simulink model "assignment_project_onclass_observerp"  (R2022a)
settings: Solver=VariableStepAuto  StartTime=0.0  StopTime=100  FixedStep=0.001  RelTol=1e-3
values from neighbouring files (symbols this model uses):
  A_LD = [  -skew(Oc),    eye(3),          -skew(Vc),      zeros(3),      zeros(3,4) ... (first row only)    [project_disturbance_observer.m]
  B_LD = [    [0;0;0],     zeros(3) ... (first row only)    [project_disturbance_observer.m]
  C_LD = [eye(3),zeros(3),zeros(3),zeros(3),zeros(3,4) ... (first row only)    [project_disturbance_observer.m]
  K = lqr(A, B, Q, R)    [Linear_model.m]    (also in project_disturbance_observer.m = lqr(A_LD,B_LD,Q,R))
undefined symbols (not defined in the file or in its folder): L
libraries: robotcorelib x1, uavutilslib x1
settings Model: PacingRate=5  Creator=yulinchen  LastModifiedBy=FLKU
settings SolverCC: AlgebraicLoopSolver=TrustRegion
settings DebuggingCC: SFMachineParentedDataDiag=warning
settings ModelReferenceCC: EnableRefExpFcnMdlSchedulingChecks=off
settings RTWCC: Description=Generic Real-Time Target

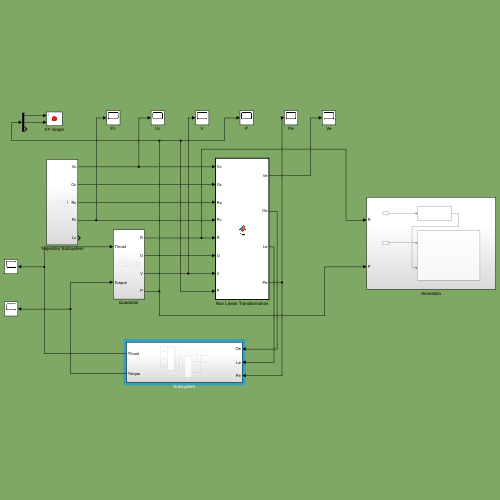
[thumbnail: Simulink's stored preview of the top-level diagram]
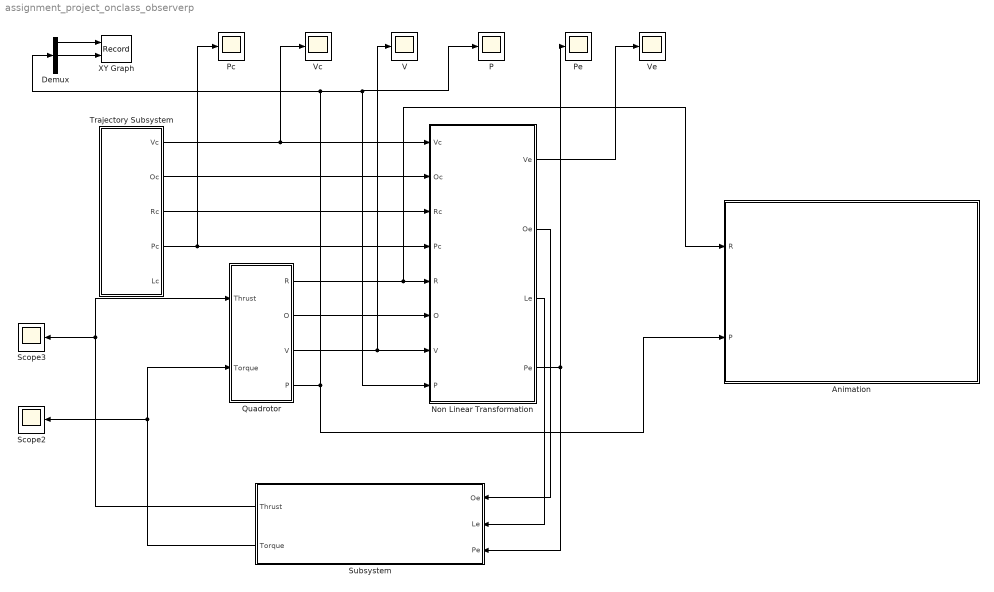
== system assignment_project_onclass_observerp ==
  Animation : Subsystem
  Demux : Demux  Outputs=3
  Non Linear Transformation : MATLAB Function  TreatAsAtomicUnit=on
  P : Scope
  Pc : Scope
  Pe : Scope
  Quadrotor : Subsystem
  Scope2 : Scope
  Scope3 : Scope
  Subsystem : Subsystem
  Trajectory Subsystem : Subsystem
  V : Scope
  Vc : Scope
  Ve : Scope
  XY Graph : Record  FileSettingsInternal="{\"entries\":[{\"content\":{\"excelSettings\":{\"content\":{},\"type\":\"Streamout.ExcelSettings\"}},\"type\":\"Streamout.FileSettingStorage\",\"uuid\":\"d99a883c-f2c1-4db8-87d8-b50552af1765\"}],\"packageUris\":[\"http://schema.mathworks.com/mf0/streamout_blocks/R2020a\"],\"version\":\"1.0\"}"  Layout=[1 1]  SignalsInternal="{\"entries\":[{\"content\":{\"signals\":[{\"content\":{\"blockPath\":[\"assignment_project_onclass_observerp/XY Graph\"],\"channel\":[],\"dimensions\":[1],\"domain\":\"assignment_project_onclass_observerp/XY Graph\",\"lineColor\":\"#a2142f\",\"plots\":[1],\"port\":1,\"sid\":[\"\"],\"signalID\":262,\"signalName\":\"Demux:1\"},\"type\":\"RecordBlkView.Signal\",\"uuid\":\"ec450a59-525e-442a-974f-52693ac6a144\"},{\"content\":{\"blockPath\":[\"assignment_project_onclass_observerp/XY Graph\"],\"channel\":[],\"dimensions\":[1],\"domain\":\"assignment_project_onclass_observerp/XY Graph\",\"lineColor\":\"#139fff\",\"plots\":[1],\"port\":2,\"sid\":[\"\"],\"signalID\":266,\"signalName\":\"Demux:2\"},\"type\":\"RecordBlkView.Signal\",\"uuid\":\"cccf172e-75eb-4d21-8fee-72d7a7188919\"}]},\"type\":\"RecordBlkView.InputSignals\",\"uuid\":\"7c770795-19c4-4b78-8178-cc713b2e03cc\"}],\"packageUris\":[\"http://schema.mathworks.com/mf0/streamout_blocks/R2020a\"],\"version\":\"1.0\"}"  VisualizationBindings="{\"xyplotplugin\":{\"info\":[{\"series\":[{\"bindingParametersList\":[{\"parameter\":\"X-Axis\",\"signalID\":262,\"signalName\":\"Demux:1\"},{\"parameter\":\"Y-Axis\",\"signalID\":266,\"signalName\":\"Demux:2\"}],\"seriesID\":13484}],\"subplotID\":1}]}}"  CompatibilityTag=XY  st=-1
  wires:
  Trajectory Subsystem/1(Vc) -> Vc/1, Non Linear Transformation/1(Vc)
  Trajectory Subsystem/2(Oc) -> Non Linear Transformation/2(Oc)
  Trajectory Subsystem/3(Rc) -> Non Linear Transformation/3(Rc)
  Trajectory Subsystem/4(Pc) -> Pc/1, Non Linear Transformation/4(Pc)
  Quadrotor/1(R) -> Animation/1(R), Non Linear Transformation/5(R)
  Quadrotor/2(O) -> Non Linear Transformation/6(O)
  Quadrotor/3(V) -> V/1, Non Linear Transformation/7(V)
  Quadrotor/4(P) -> Animation/2(P), Demux/1, Non Linear Transformation/8(P), P/1
  Non Linear Transformation/1(Ve) -> Ve/1
  Demux/1 -> XY Graph/1
  Non Linear Transformation/4(Pe) -> Pe/1, Subsystem/3(Pe)
  Subsystem/1(Thrust) -> Quadrotor/1(Thrust), Scope3/1
  Subsystem/2(Torque) -> Quadrotor/2(Torque), Scope2/1
  Non Linear Transformation/2(Oe) -> Subsystem/1(Oe)
  Non Linear Transformation/3(Le) -> Subsystem/2(Le)
  Demux/2 -> XY Graph/2

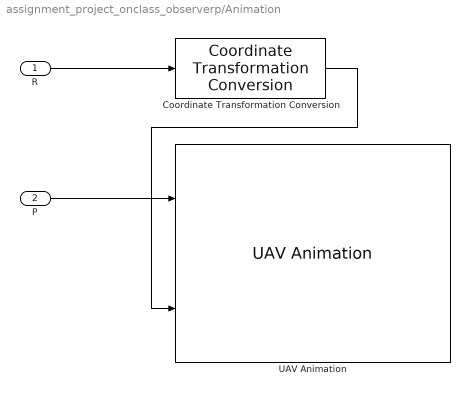
== system assignment_project_onclass_observerp/Animation ==
  R : Inport
  P : Inport  Port=2
  Coordinate Transformation Conversion : robotcorelib/Coordinate Transformation Conversion  InputRepresentation=Rotation Matrix  InputEulerSequence=ZYX  ShowTrVecInputPort=on  OutputRepresentation=Quaternion  OutputEulerSequence=ZYX  ShowTrVecOutputPort=on  SimulateUsing=Interpreted execution
      settings: SourceProductBaseCode=RO,NV,RR,UV
  UAV Animation : uavutilslib/UAV Animation  UAVType=Multirotor  UAVSize=1  InertialZDirection=Down  SampleTime=-1
      settings: SourceProductBaseCode=UV
  wires:
  Coordinate Transformation Conversion/1 -> UAV Animation/2
  P/1 -> UAV Animation/1
  R/1 -> Coordinate Transformation Conversion/1

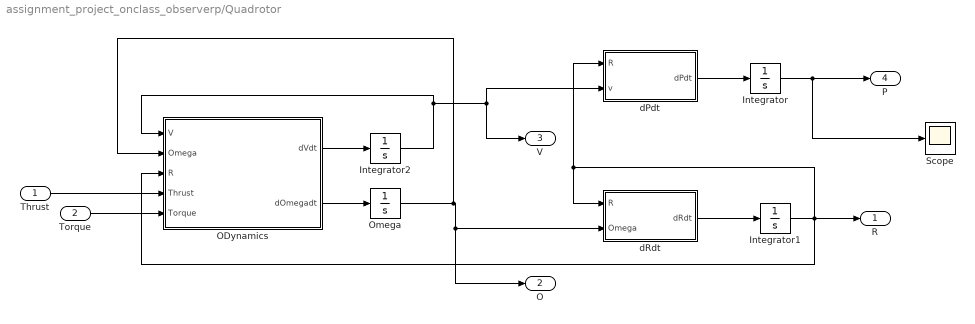
== system assignment_project_onclass_observerp/Quadrotor ==
  Thrust : Inport
  Torque : Inport  Port=2
  Integrator : Integrator  InitialCondition=[0;0;0]
  Integrator1 : Integrator  InitialCondition=eye(3)
  Integrator2 : Integrator  InitialCondition=[0;0;0]
  ODynamics : MATLAB Function  TreatAsAtomicUnit=on
  Omega : Integrator  InitialCondition=[0;0;0]
  Scope : Scope
  dPdt : MATLAB Function  TreatAsAtomicUnit=on
  dRdt : MATLAB Function  TreatAsAtomicUnit=on
  R : Outport
  O : Outport  Port=2
  V : Outport  Port=3
  P : Outport  Port=4
  wires:
  Torque/1 -> ODynamics/5(Torque)
  dRdt/1(dRdt) -> Integrator1/1
  ODynamics/2(dOmegadt) -> Omega/1
  Integrator2/1 -> ODynamics/1(V), V/1, dPdt/2(v)
  Thrust/1 -> ODynamics/4(Thrust)
  Integrator1/1 -> ODynamics/3(R), dRdt/1(R), dPdt/1(R), R/1
  dPdt/1(dPdt) -> Integrator/1
  Omega/1 -> ODynamics/2(Omega), O/1, dRdt/2(Omega)
  Integrator/1 -> Scope/1, P/1
  ODynamics/1(dVdt) -> Integrator2/1

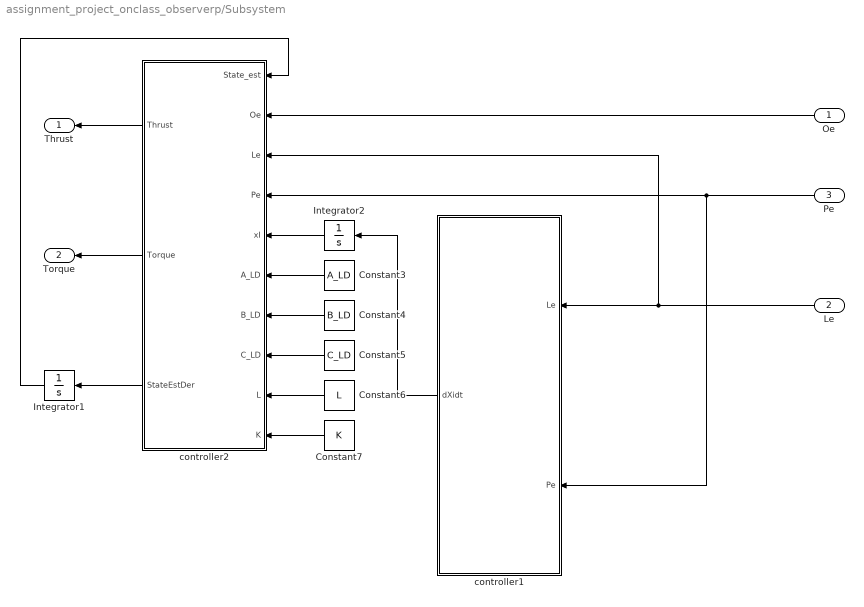
== system assignment_project_onclass_observerp/Subsystem ==
  Oe : Inport
  Le : Inport  Port=2
  Pe : Inport  Port=3
  Constant3 : Constant  Value=A_LD
  Constant4 : Constant  Value=B_LD
  Constant5 : Constant  Value=C_LD
  Constant6 : Constant  Value=L
  Constant7 : Constant  Value=K
  Integrator1 : Integrator  InitialCondition=[0;0;0;0;0;0;0;0;0;0;0;0;0;0;0;0]
  Integrator2 : Integrator  InitialCondition=[0;0;0;0]
  controller1 : MATLAB Function  TreatAsAtomicUnit=on
  controller2 : MATLAB Function  TreatAsAtomicUnit=on
  Thrust : Outport
  Torque : Outport  Port=2
  wires:
  Integrator1/1 -> controller2/1(State_est)
  Le/1 -> controller2/3(Le), controller1/1(Le)
  Integrator2/1 -> controller2/5(xI)
  Constant5/1 -> controller2/8(C_LD)
  Constant6/1 -> controller2/9(L)
  Constant7/1 -> controller2/10(K)
  Pe/1 -> controller1/2(Pe), controller2/4(Pe)
  controller2/3(StateEstDer) -> Integrator1/1
  Constant3/1 -> controller2/6(A_LD)
  Constant4/1 -> controller2/7(B_LD)
  controller1/1(dXidt) -> Integrator2/1
  controller2/2(Torque) -> Torque/1
  controller2/1(Thrust) -> Thrust/1
  Oe/1 -> controller2/2(Oe)

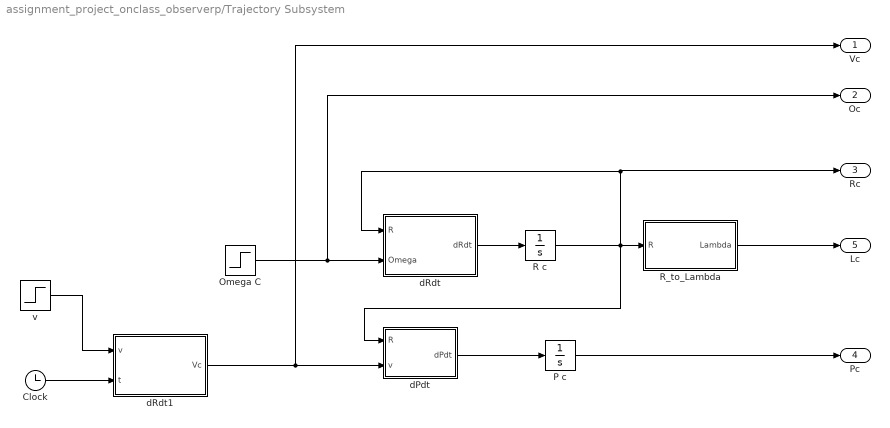
== system assignment_project_onclass_observerp/Trajectory Subsystem ==
  Clock : Clock
  Omega C : Step  Time=0  Before=[0;0;0]  After=[0;0;0]  SampleTime=0
  P c : Integrator
  R c : Integrator  InitialCondition=eye(3)
  "R_to_Lambda " : MATLAB Function  TreatAsAtomicUnit=on
  dPdt : MATLAB Function  TreatAsAtomicUnit=on
  dRdt : MATLAB Function  TreatAsAtomicUnit=on
  dRdt1 : MATLAB Function  TreatAsAtomicUnit=on
  v : Step  Time=0  Before=0.25  After=0.25  SampleTime=0
  Vc : Outport
  Oc : Outport  Port=2
  Rc : Outport  Port=3
  Pc : Outport  Port=4
  Lc : Outport  Port=5
  wires:
  Omega C/1 -> Oc/1, dRdt/2(Omega)
  R c/1 -> Rc/1, dRdt/1(R), "R_to_Lambda "/1(R), dPdt/1(R)
  "R_to_Lambda "/1(Lambda) -> Lc/1
  P c/1 -> Pc/1
  dRdt1/1(Vc) -> Vc/1, dPdt/2(v)
  dPdt/1(dPdt) -> P c/1
  dRdt/1(dRdt) -> R c/1
  Clock/1 -> dRdt1/2(t)
  v/1 -> dRdt1/1(v)

== matlab function assignment_project_onclass_observerp/Subsystem/controller1 ==
  data: Le input; Pe input; dXidt output
function dXidt= Instates(Le,Pe)

dXidt=[Pe;Le(3)];


end

== matlab function assignment_project_onclass_observerp/Subsystem/controller2 ==
  data: State_est input; Oe input; Le input; Pe input; Thrust output; Torque output; xI input; A_LD input; B_LD input; C_LD input; L input; K input; StateEstDer output
function [Thrust,Torque,StateEstDer]= ctrlObserver(State_est,Oe,Le,Pe,xI,A_LD,B_LD,C_LD,L,K)
%dx=[dPe,dVe,dLe,dOe,xI]
u=-K*State_est;
y=[Pe;Le;Oe;xI];
StateEstDer=(A_LD-L*C_LD)*State_est+L*y+B_LD*u;
Thrust=u(1);
Torque=u(2:4);

end

== matlab function assignment_project_onclass_observerp/Trajectory Subsystem/dPdt ==
  data: R input; dPdt output; v input
function dPdt = fcn(R,v)
dPdt=R*v;
end

== matlab function assignment_project_onclass_observerp/Trajectory Subsystem/dRdt ==
  data: R input; dRdt output; Omega input
function dRdt = fcn(R,Omega)

dRdt=R*skew(Omega);

end

== matlab function assignment_project_onclass_observerp/Trajectory Subsystem/R_to_Lambda  ==
  data: R input; Lambda output
function Lambda = fcn(R)


Pitch=atan2(-R(3,1),sqrt(R(1,1)^2+R(2,1)^2));
Yaw=atan2(R(2,1)/cos(Pitch),R(1,1)/cos(Pitch));
Roll=atan2(R(3,2)/cos(Pitch),R(3,3)/cos(Pitch));
Lambda=[Roll,Pitch,Yaw];

end

== matlab function assignment_project_onclass_observerp/Quadrotor/ODynamics ==
  data: V input; Omega input; R input; dVdt output; Thrust input; Torque input; dOmegadt output
function [dVdt,dOmegadt]= fcn(V,Omega,R,Thrust,Torque)
m=0.25;
g=9.8;

J=[10^-1,0,0;0,10^-1,0;0,0,10^-1];

dVdt=-skew(Omega)*V-1/m*([0;0;Thrust])+R'*[0;0;g]+R'*[m*0.1;0;0];
dOmegadt=-J^-1*skew(Omega)*J*Omega+J^-1*Torque;
end

== matlab function assignment_project_onclass_observerp/Quadrotor/dRdt ==
  data: R input; dRdt output; Omega input
function dRdt = fcn(R,Omega)

dRdt=R*skew(Omega);
end

== matlab function assignment_project_onclass_observerp/Quadrotor/dPdt ==
  data: R input; dPdt output; v input
function dPdt = fcn(R,v)

dPdt=R*v;

end

== matlab function assignment_project_onclass_observerp/Non Linear Transformation ==
  data: Vc input; Oc input; Rc input; Pc input; R input; O input; V input; Ve output; P input; Oe output; Le output; Pe output
function [Ve,Oe,Le,Pe]= fcn(Vc,Oc,Rc,Pc,R,O,V,P)

Ve=V-Vc;
Oe=O-Oc;
Re=R*Rc';
Pitch=atan2(-Re(3,1),sqrt(Re(1,1)^2+Re(2,1)^2));
Yaw=atan2(Re(2,1)/cos(Pitch),Re(1,1)/cos(Pitch));
Roll=atan2(Re(3,2)/cos(Pitch),Re(3,3)/cos(Pitch));
Le=[Roll;Pitch;Yaw];
Pe=P-Pc;


end

== matlab function assignment_project_onclass_observerp/Trajectory Subsystem/dRdt1 ==
  data: v input; Vc output; t input
function Vc=VcGen(v,t)
Vc=[0;0;0];
if (t>20)
    Vc=[v;0;0]; %  vm/s  along x
end
if (t>28)
    Vc=[0;v;0];  %-vm/s  along y
end
if (t>36)
    Vc=[-v;0;0];%   vm/s  along x
end

if (t>44)
    Vc=[0;-v;0];%   -vm/s  along y
end

if (t>60)
    Vc=[0;0;0];%   -vm/s  along y
end
end
